simulink model "Graficas_simulink"  (R2020a)
settings: Solver=VariableStepAuto  StartTime=0.0  StopTime=147  RelTol=1e-3
settings Model: Creator=HP  LastModifiedBy=HP

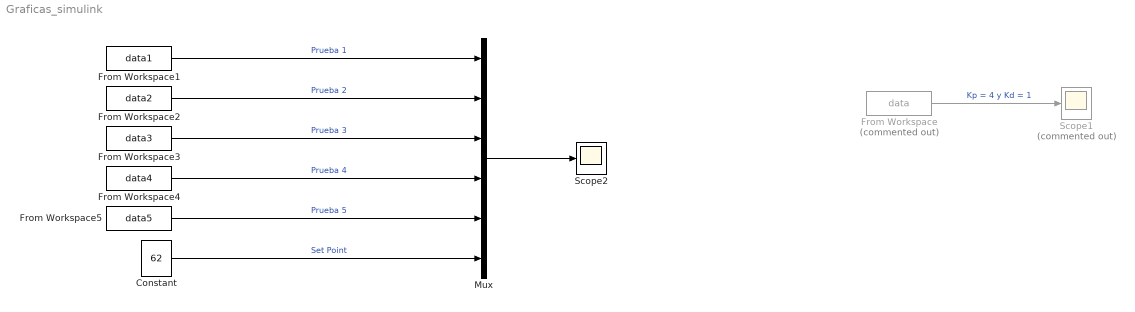
== system Graficas_simulink ==
  Constant : Constant  Value=62
  From Workspace : FromWorkspace  Commented=on  VariableName=data
  From Workspace1 : FromWorkspace  VariableName=data1
  From Workspace2 : FromWorkspace  VariableName=data2
  From Workspace3 : FromWorkspace  VariableName=data3
  From Workspace4 : FromWorkspace  VariableName=data4
  From Workspace5 : FromWorkspace  VariableName=data5
  Mux : Mux  Inputs=6
  Scope1 : Scope  Commented=on
  Scope2 : Scope
  wires:
  From Workspace/1 -> Scope1/1  "Kp = 4 y Kd = 1"
  Mux/1 -> Scope2/1
  From Workspace1/1 -> Mux/1  "Prueba 1"
  From Workspace2/1 -> Mux/2  "Prueba 2"
  From Workspace3/1 -> Mux/3  "Prueba 3"
  From Workspace4/1 -> Mux/4  "Prueba 4"
  From Workspace5/1 -> Mux/5  "Prueba 5"
  Constant/1 -> Mux/6  "Set Point"
